simulink model "Traction_Control"  (R2025b)
settings: Solver=VariableStepAuto  StartTime=0.0  StopTime=10.0  RelTol=1e-3
model workspace (MAT data in the model file):
  fz_values = [0 50 100 150 200 250 300 350 400 450 500 550 600 650 700 750 800 850 900 950 1000 1050 1100 1150 1200 1250 1300 1350 1400 1450 1500 1550 1600 1650 1700 1750 1800 1850 1900 1950 2000 2050 2100]
  k_opt_lut = [0 0 0 0 0 0 0 0 0 0 0 0 ... (4386 elements, 51x2x43)]
  mu_opt_lut = [0 0 0 0 0 0 0 0 0 0 0 0 ... (4386 elements, 51x2x43)]
libraries: slpidlib x1, simulink x1
(part 1 of 2)
settings Model: Creator=benjaminlevin  LastModifiedBy=benjaminlevin

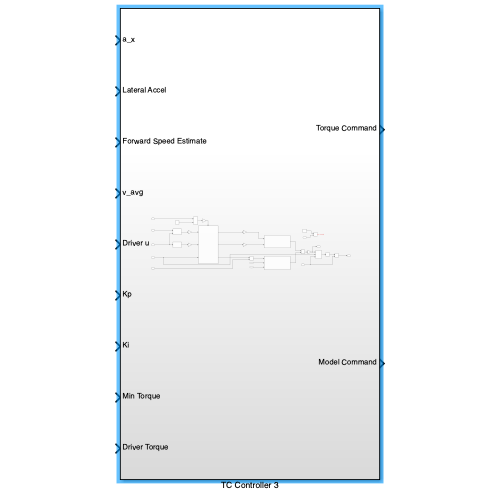
[thumbnail: Simulink's stored preview of the top-level diagram]
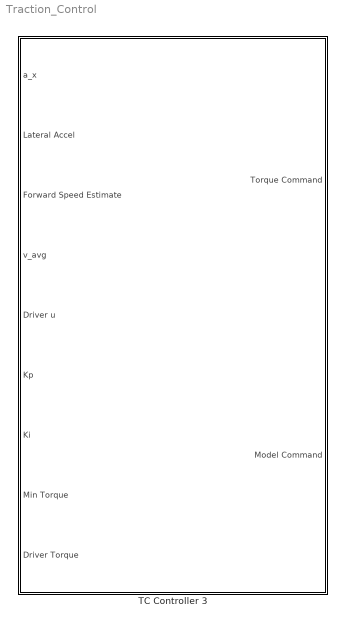
== system Traction_Control ==
  TC Controller 3 : Subsystem

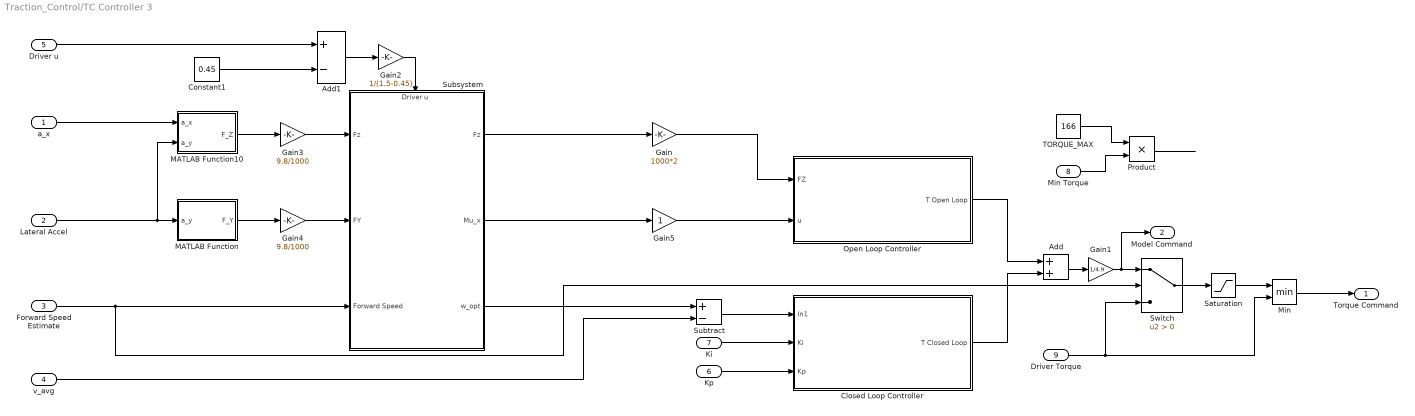
== system Traction_Control/TC Controller 3 ==
  a_x : Inport
  Lateral Accel : Inport  Port=2
  Forward Speed Estimate : Inport  Port=3
  v_avg : Inport  Port=4
  Driver u : Inport  Port=5
  Kp : Inport  Port=6
  Ki : Inport  Port=7
  Min Torque : Inport  Port=8
  Driver Torque : Inport  Port=9
  Add : Sum
  Add1 : Sum  Inputs=+-
  Closed Loop Controller : Subsystem
  Constant1 : Constant  Value=0.45
  Gain : Gain  Gain=1000*2
  Gain1 : Gain  Gain=1/4.9
  Gain2 : Gain  Gain=1/(1.5-0.45)
  Gain3 : Gain  Gain=9.8/1000
  Gain4 : Gain  Gain=9.8/1000
  Gain5 : Gain
  MATLAB Function : MATLAB Function  TreatAsAtomicUnit=on
  MATLAB Function10 : MATLAB Function  TreatAsAtomicUnit=on
  Min : MinMax  Inputs=2
  Open Loop Controller : Subsystem
  Product : Product
  Saturation : Saturate  UpperLimit=166  LowerLimit=0
  Subsystem : Subsystem
      settings: PortSchema="{\"entries\":[{\"content\":{\"sides\":[{\"content\":{\"connectorIds\":[\"In1\",\"In2\",\"In3\"]},\"type\":\"ConnectorPlacement.EquallySpacedRectSide\",\"uuid\":\"52cb1509-e05e-4bae-af08-b3cbe80ce8d7\"},{\"content\":{\"connectorIds\":[\"Out1\",\"Out2\",\"Out3\"],\"side\":\"RIGHT\"},\"type\":\"ConnectorPlacement.EquallySpacedRectSide\",\"uuid\":\"5c1b6c4d-f36b-4262-971d-310d950de965\"},{\"content\":{\"connectorIds\":[\"In4\"],\"side\":\"TOP\"},\"type\":\"ConnectorPlacement.EquallySpacedRectSide\",\"uuid\":\"90df2961-afb4-4b60-bc78-aaa8af520e7a\"}]},\"type\":\"ConnectorPlacement.EquallySpacedConnector\",\"uuid\":\"073ed346-9857-4a79-b76f-e1da7d32971a\"}],\"packageUris\":[\"http://schema.mathworks.com/mf0/Connector/R2020b\"],\"version\":\"1.0\"}"
  Subtract : Sum  Inputs=+-
  Switch : Switch  Criteria=u2 > Threshold  SaturateOnIntegerOverflow=off  InputSameDT=off
  TORQUE_MAX : Constant  Value=166
  Torque Command : Outport
  Model Command : Outport  Port=2
  wires:
  Gain1/1 -> Model Command/1, Switch/1
  MATLAB Function10/1(F_Z) -> Gain3/1
  Open Loop Controller/1(T Open Loop) -> Add/1
  Add/1 -> Gain1/1
  v_avg/1 -> Subtract/2
  Kp/1 -> Closed Loop Controller/3(Kp)
  Forward Speed Estimate/1 -> Switch/2, Subsystem/3(Forward Speed)
  Driver Torque/1 -> Switch/3, Min/2
  Ki/1 -> Closed Loop Controller/2(Ki)
  TORQUE_MAX/1 -> Product/1
  Min Torque/1 -> Product/2
  Lateral Accel/1 -> MATLAB Function10/2(a_y), MATLAB Function/1(a_y)
  Driver u/1 -> Add1/1
  Constant1/1 -> Add1/2
  Add1/1 -> Gain2/1
  Gain2/1 -> Subsystem/4(Driver u)
  Subsystem/3(w_opt) -> Subtract/1
  Subsystem/1(Fz) -> Gain/1
  Subsystem/2(Mu_x) -> Gain5/1
  Gain4/1 -> Subsystem/2(FY)
  MATLAB Function/1(F_Y) -> Gain4/1
  Gain3/1 -> Subsystem/1("Fz ")
  a_x/1 -> MATLAB Function10/1(a_x)
  Gain/1 -> Open Loop Controller/1(FZ)
  Gain5/1 -> Open Loop Controller/2(u)
  Subtract/1 -> Closed Loop Controller/1(In1)
  Saturation/1 -> Min/1
  Switch/1 -> Saturation/1
  Product/1 -> ?
  Closed Loop Controller/1(T Closed Loop) -> Add/2
  Min/1 -> Torque Command/1

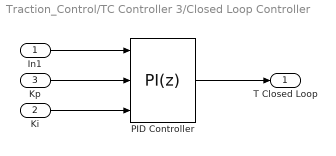
== system Traction_Control/TC Controller 3/Closed Loop Controller ==
  In1 : Inport
  Ki : Inport  Port=2
  Kp : Inport  Port=3
  PID Controller : slpidlib/PID Controller  Controller=PI  Form=Parallel  TimeDomain=Discrete-time  UseExternalTs=off  SampleTime=-1  IntegratorMethod=Forward Euler  FilterMethod=Forward Euler  ControllerParametersSource=external  P=100  I=10  UseKiTs=off  D=0  UseExternalDerivativeSource=off  N=100  UseFilter=on  TunerSelectOption=Transfer Function Based (PID Tuner App)  InitialConditionSource=internal  InitialConditionForIntegrator=0  InitialConditionForFilter=0  DifferentiatorICPrevScaledInput=0  ExternalReset=none  TrackingMode=off  Kt=1  LimitOutput=on  SatLimitsSource=internal  UpperSaturationLimit=166*4.9  LowerSaturationLimit=-166*4.9  LinearizeAsGain=on  AntiWindupMode=clamping  Kb=1  LimitIntegrator=on  UpperIntegratorSaturationLimit=166*4.9  LowerIntegratorSaturationLimit=-166*4.9  POutMin=[]  POutMax=[]  IOutMin=[]  IOutMax=[]  DOutMin=[]  DOutMax=[]  NOutMin=[]  NOutMax=[]  SumOutMin=[]  SumOutMax=[]  SaturationOutMin=[]  SaturationOutMax=[]  PParamMin=[]  PParamMax=[]  IParamMin=[]  IParamMax=[]  DParamMin=[]  DParamMax=[]  NParamMin=[]  NParamMax=[]  KbParamMin=[]  KbParamMax=[]  KtParamMin=[]  KtParamMax=[]  KbOutMin=[]  KbOutMax=[]  KtOutMin=[]  KtOutMax=[]  IntegratorOutMin=[]  IntegratorOutMax=[]  FilterOutMin=[]  FilterOutMax=[]  SumI1OutMin=[]  SumI1OutMax=[]  SumI2OutMin=[]  SumI2OutMax=[]  SumI3OutMin=[]  SumI3OutMax=[]  SumI4OutMin=[]  SumI4OutMax=[]  SumDOutMin=[]  SumDOutMax=[]  DifferentiatorOutMin=[]  DifferentiatorOutMax=[]  FilterDiffOutCoefMin=[]  FilterDiffOutCoefMax=[]  ReciprocalOutMin=[]  ReciprocalOutMax=[]  SumDenOutMin=[]  SumDenOutMax=[]  SumNumOutMin=[]  SumNumOutMax=[]  DivideOutMin=[]  DivideOutMax=[]  UdiffTsProdOutMin=[]  UdiffTsProdOutMax=[]  NTsProdOutMin=[]  NTsProdOutMax=[]  UintegralTsProdOutMin=[]  UintegralTsProdOutMax=[]  UngainTsProdOutMin=[]  UngainTsProdOutMax=[]  ClampingZeroOutDataTypeStr=Inherit: Inherit via back propagation  ClampingZeroOutMin=[]  ClampingZeroOutMax=[]  FilterDenConstantOutDataTypeStr=Inherit: Inherit via back propagation  FilterDenConstantOutMin=[]  FilterDenConstantOutMax=[]  PCopyOutDataTypeStr=Inherit: Inherit via back propagation  PCopyOutMin=[]  PCopyOutMax=[]  NCopyOutDataTypeStr=Inherit: Inherit via back propagation  NCopyOutMin=[]  NCopyOutMax=[]  IntegratorContinuousStateAttributes=''  IntegratorStateMustResolveToSignalObject=off  IntegratorRTWStateStorageClass=Auto  FilterContinuousStateAttributes=''  FilterStateMustResolveToSignalObject=off  FilterRTWStateStorageClass=Auto  ParallelPVariant=ExternalParameters  IdealPVariant=Disabled  IVariant=ExternalParameters  DVariant=Disabled  IntegratorVariant=Discrete  SatVariant=Enabled  AWVariant=DiscClampingParallel  PCopyVariant=Disabled  TRVariant=Disabled  FdbkBlocksVariant=Forward  IdealPFdbkVariant=Disabled  SatFdbkVariant=Disabled  DerivativeFilterVariant=Disabled  NVariant=Disabled  NCopyVariant=Disabled_SignalSpec  FilterICVariant=Disabled  IntegratorICVariant=InternalICs  ExternalResetVariant=Disabled  TRSumVariant=Passthrough  SumFdbkVariant=Disabled  SumVariant=Sum_PI  TsampFilterVariant=InternalTs  TsampNgainVariant=Passthrough  TsampIntegralVariant=Disabled_SignalSpec  ExternalSaturationOutDataTypeStr=Inherit: Same as second input  DerivativeSourceVariant=Disabled  PreIntVariant=InternalPreInt
  T Closed Loop : Outport
  wires:
  In1/1 -> PID Controller/1
  PID Controller/1 -> T Closed Loop/1
  Kp/1 -> PID Controller/2
  Ki/1 -> PID Controller/3

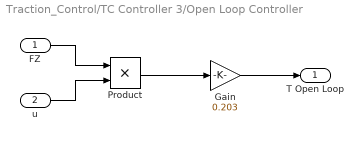
== system Traction_Control/TC Controller 3/Open Loop Controller ==
  FZ : Inport
  u : Inport  Port=2
  Gain : Gain  Gain=0.203
  Product : Product
  T Open Loop : Outport
  wires:
  FZ/1 -> Product/1
  u/1 -> Product/2
  Gain/1 -> T Open Loop/1
  Product/1 -> Gain/1
